simulink model "EIG"  (R2025b)
settings: Solver=VariableStepAuto  StartTime=0.0  StopTime=10.0  RelTol=1e-3
undefined symbols (not defined in the file): A, B, K_eig, X0
settings Model: Creator=salvo  LastModifiedBy=salvo

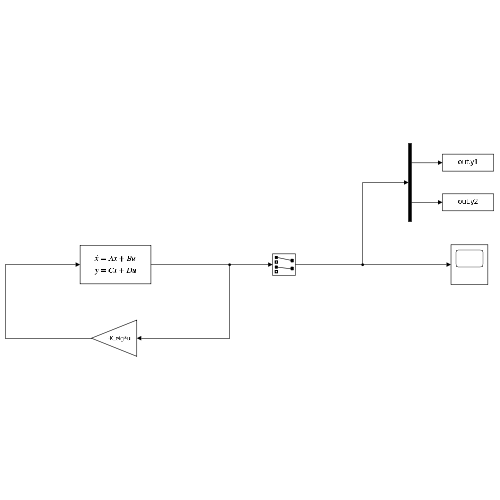
[thumbnail: Simulink's stored preview of the top-level diagram]
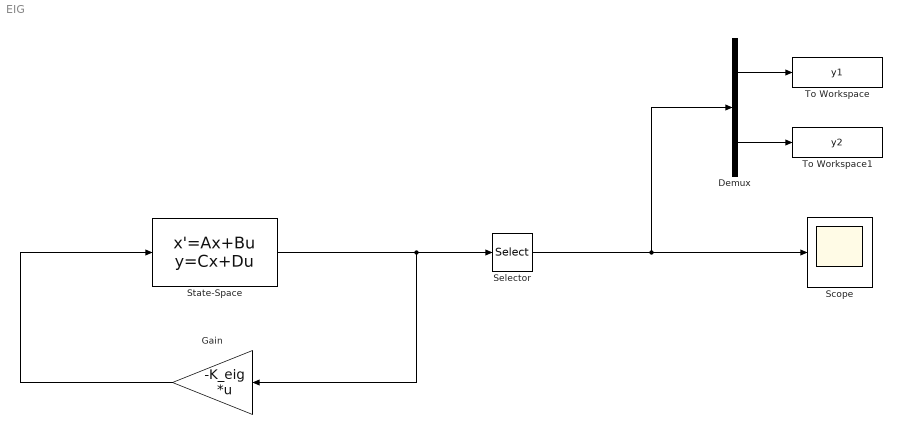
== system EIG ==
  Demux : Demux  Outputs=2
  Gain : Gain  Gain=-K_eig  Multiplication=Matrix(K*u)
  Scope : Scope
      settings: ActiveDisplayYMinimum=-0.11157378413839716  ActiveDisplayYMaximum=0.30670402359294413
  Selector : Selector  InputPortWidth=4  IndexOptions=Index vector (dialog)  Indices=[1 3]  OutputSizes=1
  State-Space : StateSpace  A=A  B=B  C=eye(4)  D=zeros(4,1)  InitialCondition=X0
  To Workspace : ToWorkspace  VariableName=y1  SaveFormat=Timeseries  SampleTime=-1
  To Workspace1 : ToWorkspace  VariableName=y2  SaveFormat=Timeseries  SampleTime=-1
  wires:
  Gain/1 -> State-Space/1
  State-Space/1 -> Gain/1, Selector/1
  Selector/1 -> Demux/1, Scope/1
  Demux/2 -> To Workspace1/1
  Demux/1 -> To Workspace/1
